simulink model "actuationModel"  (R2023a)
settings: Solver=ode1  StartTime=t0  StopTime=tfinal  FixedStep=dt  RelTol=1e-3
values from neighbouring files (symbols this model uses):
  dampCoef = 5.0    (= 5)    [actuatorControlOptimization.m]
  Iaxis = 0.05    [actuatorControlOptimization.m]
  inpAmp = 50*pi/180    (= 0.872664625997)    [actuatorControlOptimization.m]
  inpPeriod = 2    [actuatorControlOptimization.m]
  inpPhaseDelay = 1    [actuatorControlOptimization.m]
  inpPulseWidth = 50    [actuatorControlOptimization.m]
  Kd = 39.3151    [actuatorControlOptimization.m]    (also in costFunc.m = Inp(3))
  Ki = 191.1087    [actuatorControlOptimization.m]    (also in costFunc.m = Inp(2))
  Kp = 654.2698    [actuatorControlOptimization.m]    (also in costFunc.m = Inp(1))
libraries: slpidlib x1
settings Model: Creator=cmonti  LastModifiedBy=cmonti
settings DataIOCC: ReturnWorkspaceOutputsName=simout

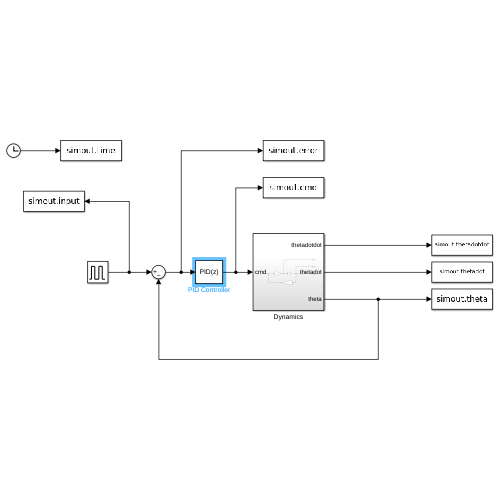
[thumbnail: Simulink's stored preview of the top-level diagram]
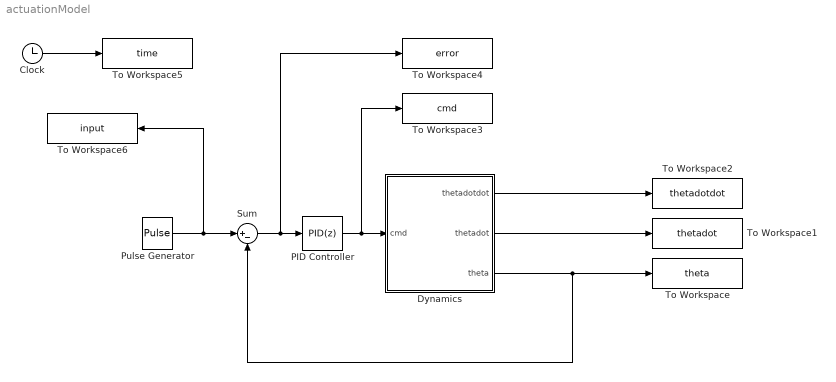
== system actuationModel ==
  Clock : Clock
  Dynamics : Subsystem
  PID Controller : slpidlib/PID Controller  Controller=PID  Form=Parallel  TimeDomain=Discrete-time  UseExternalTs=off  SampleTime=-1  IntegratorMethod=Forward Euler  FilterMethod=Forward Euler  ControllerParametersSource=internal  P=Kp  I=Ki  UseKiTs=off  D=Kd  N=100  UseFilter=on  TunerSelectOption=Transfer Function Based (PID Tuner App)  InitialConditionSource=internal  InitialConditionForIntegrator=0  InitialConditionForFilter=0  DifferentiatorICPrevScaledInput=0  ExternalReset=none  TrackingMode=off  Kt=1  LimitOutput=off  SatLimitsSource=internal  UpperSaturationLimit=inf  LowerSaturationLimit=-inf  LinearizeAsGain=on  AntiWindupMode=none  Kb=1  LimitIntegrator=off  UpperIntegratorSaturationLimit=inf  LowerIntegratorSaturationLimit=-inf  POutMin=[]  POutMax=[]  IOutMin=[]  IOutMax=[]  DOutMin=[]  DOutMax=[]  NOutMin=[]  NOutMax=[]  SumOutMin=[]  SumOutMax=[]  SaturationOutMin=[]  SaturationOutMax=[]  PParamMin=[]  PParamMax=[]  IParamMin=[]  IParamMax=[]  DParamMin=[]  DParamMax=[]  NParamMin=[]  NParamMax=[]  KbParamMin=[]  KbParamMax=[]  KtParamMin=[]  KtParamMax=[]  KbOutMin=[]  KbOutMax=[]  KtOutMin=[]  KtOutMax=[]  IntegratorOutMin=[]  IntegratorOutMax=[]  FilterOutMin=[]  FilterOutMax=[]  SumI1OutMin=[]  SumI1OutMax=[]  SumI2OutMin=[]  SumI2OutMax=[]  SumI3OutMin=[]  SumI3OutMax=[]  SumI4OutMin=[]  SumI4OutMax=[]  SumDOutMin=[]  SumDOutMax=[]  DifferentiatorOutMin=[]  DifferentiatorOutMax=[]  FilterDiffOutCoefMin=[]  FilterDiffOutCoefMax=[]  ReciprocalOutMin=[]  ReciprocalOutMax=[]  SumDenOutMin=[]  SumDenOutMax=[]  SumNumOutMin=[]  SumNumOutMax=[]  DivideOutMin=[]  DivideOutMax=[]  UdiffTsProdOutMin=[]  UdiffTsProdOutMax=[]  NTsProdOutMin=[]  NTsProdOutMax=[]  UintegralTsProdOutMin=[]  UintegralTsProdOutMax=[]  UngainTsProdOutMin=[]  UngainTsProdOutMax=[]  ClampingZeroOutDataTypeStr=Inherit: Inherit via back propagation  ClampingZeroOutMin=[]  ClampingZeroOutMax=[]  FilterDenConstantOutDataTypeStr=Inherit: Inherit via back propagation  FilterDenConstantOutMin=[]  FilterDenConstantOutMax=[]  PCopyOutDataTypeStr=Inherit: Inherit via back propagation  PCopyOutMin=[]  PCopyOutMax=[]  NCopyOutDataTypeStr=Inherit: Inherit via back propagation  NCopyOutMin=[]  NCopyOutMax=[]  IntegratorContinuousStateAttributes=''  IntegratorStateMustResolveToSignalObject=off  IntegratorRTWStateStorageClass=Auto  FilterContinuousStateAttributes=''  FilterStateMustResolveToSignalObject=off  FilterRTWStateStorageClass=Auto  ParallelPVariant=InternalParameters  IdealPVariant=Disabled  IVariant=InternalParameters  DVariant=InternalParameters  IntegratorVariant=Discrete  SatVariant=Disabled  AWVariant=Passthrough  PCopyVariant=Disabled  TRVariant=Disabled  FdbkBlocksVariant=Forward  IdealPFdbkVariant=Disabled  SatFdbkVariant=Disabled  DerivativeFilterVariant=ForwardEulerFilter  NVariant=InternalParameters  NCopyVariant=Disabled  FilterICVariant=InternalICsFilter  IntegratorICVariant=InternalICs  ExternalResetVariant=Disabled  TRSumVariant=Passthrough  SumFdbkVariant=Disabled  SumVariant=Sum_PID  TsampFilterVariant=InternalTs  TsampNgainVariant=Passthrough  TsampIntegralVariant=Disabled_SignalSpec  ExternalSaturationOutDataTypeStr=Inherit: Same as second input
  Pulse Generator : DiscretePulseGenerator  PulseType=Time based  Amplitude=inpAmp  Period=inpPeriod  PulseWidth=inpPulseWidth  PhaseDelay=inpPhaseDelay
  Sum : Sum  Inputs=|+-
  To Workspace : ToWorkspace  VariableName=theta  SampleTime=-1
  To Workspace1 : ToWorkspace  VariableName=thetadot  SampleTime=-1
  To Workspace2 : ToWorkspace  VariableName=thetadotdot  SampleTime=-1
  To Workspace3 : ToWorkspace  VariableName=cmd  SampleTime=-1
  To Workspace4 : ToWorkspace  VariableName=error  SampleTime=-1
  To Workspace5 : ToWorkspace  VariableName=time  SampleTime=-1
  To Workspace6 : ToWorkspace  VariableName=input  SampleTime=-1
  wires:
  Dynamics/1(thetadotdot) -> To Workspace2/1
  Dynamics/2(thetadot) -> To Workspace1/1
  Dynamics/3(theta) -> Sum/2, To Workspace/1
  Pulse Generator/1 -> To Workspace6/1, Sum/1
  PID Controller/1 -> To Workspace3/1, Dynamics/1(cmd)
  Sum/1 -> To Workspace4/1, PID Controller/1
  Clock/1 -> To Workspace5/1

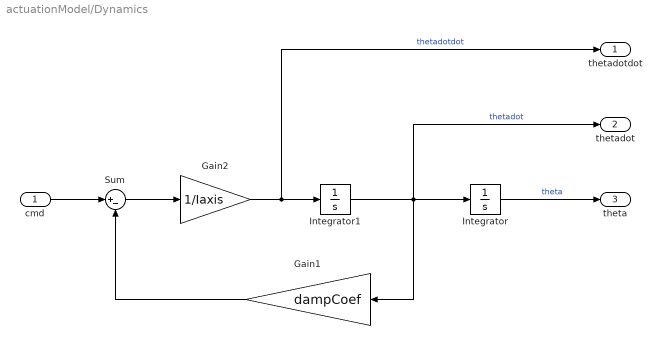
== system actuationModel/Dynamics ==
  cmd : Inport
  Gain1 : Gain  Gain=dampCoef
  Gain2 : Gain  Gain=1/Iaxis
  Integrator : Integrator  WrapState=on
  Integrator1 : Integrator
  Sum : Sum  Inputs=|+-
  thetadotdot : Outport
  thetadot : Outport  Port=2
  theta : Outport  Port=3
  wires:
  Gain1/1 -> Sum/2
  Integrator1/1 -> thetadot/1, Integrator/1, Gain1/1  "thetadot"
  cmd/1 -> Sum/1
  Integrator/1 -> theta/1  "theta"
  Sum/1 -> Gain2/1
  Gain2/1 -> thetadotdot/1, Integrator1/1  "thetadotdot"
